simulink model "MagLevNL_wNoise_Lab10_CS"  (Simulink 10.0)
settings: Solver=VariableStepAuto  StartTime=0.0  StopTime=30  MaxStep=1e-4  RelTol=1e-6  AbsTol=1e-6
InitFcn:
  | K_plant = 1.241578125e-3+0.3*(1-2*rand)*1e-3
libraries: cstblocks x1, simulink x1
settings Model: Creator=MENGQI  LastModifiedBy=Santoshi Kulkarni
settings SolverCC: AutoScaleAbsTol=off  InitialStep=1e-7
settings DataIOCC: SaveFormat=Dataset
settings OptimizationCC: LifeSpan=auto
settings DebuggingCC: UnderspecifiedInitializationDetection=Simplified  MergeDetectMultiDrivingBlocksExec=error  SFUnexpectedBacktrackingDiag=error  SFNoUnconditionalDefaultTransitionDiag=error  SFExecutionAtInitializationDiag=warning
settings HardwareCC: ProdBitPerPointer=64  ProdBitPerSizeT=64  ProdBitPerPtrDiffT=64  ProdLargestAtomicFloat=Float  ProdIntDivRoundTo=Zero  ProdEndianess=LittleEndian  ProdWordSize=64  ProdHWDeviceType=Intel->x86-64 (Windows64)
settings ModelReferenceCC: PropagateSignalLabelsOutOfModel=on
settings GRTTargetCC: TargetLangStandard=C99 (ISO)  CombineOutputUpdateFcns=on  GRTInterface=off
settings ConfigComp: CovMetricSettings=dwe  CovHtmlReporting=off  CovSaveCumulativeToWorkspaceVar=off  CovSaveSingleToWorkspaceVar=off

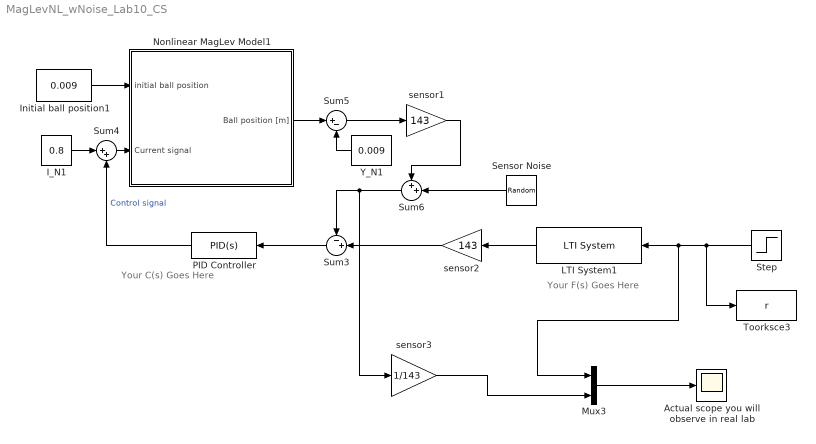
== system MagLevNL_wNoise_Lab10_CS ==
  note: Your F(s) Goes Here
  note: Your C(s) Goes Here
  Actual scope you will observe in real lab : Scope
  I_N1 : Constant  Value=0.8
  Initial ball position1 : Constant  Value=0.009
  LTI System1 : cstblocks/LTI System  sys=tf(5,[1 5])  IC=[]
  Mux3 : Mux  Inputs=2
  Nonlinear MagLev Model1 : Subsystem
  PID Controller : simulink/Continuous/PID Controller  Controller=PID  Form=Parallel  TimeDomain=Continuous-time  SampleTime=-1  IntegratorMethod=Forward Euler  FilterMethod=Forward Euler  ControllerParametersSource=internal  P=-4.45  I=-3.09  D=-0.0532  UseFilter=on  N=1000  TunerSelectOption=Transfer Function Based (PID Tuner App)  InitialConditionSource=internal  InitialConditionForIntegrator=0  InitialConditionForFilter=0  DifferentiatorICPrevScaledInput=0  ExternalReset=none  TrackingMode=off  Kt=1  LimitOutput=off  UpperSaturationLimit=inf  LowerSaturationLimit=-inf  LinearizeAsGain=on  AntiWindupMode=none  Kb=1  POutMin=[]  POutMax=[]  IOutMin=[]  IOutMax=[]  DOutMin=[]  DOutMax=[]  NOutMin=[]  NOutMax=[]  SumOutMin=[]  SumOutMax=[]  SaturationOutMin=[]  SaturationOutMax=[]  PParamMin=[]  PParamMax=[]  IParamMin=[]  IParamMax=[]  DParamMin=[]  DParamMax=[]  NParamMin=[]  NParamMax=[]  KbParamMin=[]  KbParamMax=[]  KtParamMin=[]  KtParamMax=[]  KbOutMin=[]  KbOutMax=[]  KtOutMin=[]  KtOutMax=[]  IntegratorOutMin=[]  IntegratorOutMax=[]  FilterOutMin=[]  FilterOutMax=[]  SumI1OutMin=[]  SumI1OutMax=[]  SumI2OutMin=[]  SumI2OutMax=[]  SumI3OutMin=[]  SumI3OutMax=[]  SumI4OutMin=[]  SumI4OutMax=[]  SumDOutMin=[]  SumDOutMax=[]  DifferentiatorOutMin=[]  DifferentiatorOutMax=[]  FilterDiffOutCoefMin=[]  FilterDiffOutCoefMax=[]  ReciprocalOutMin=[]  ReciprocalOutMax=[]  SumDenOutMin=[]  SumDenOutMax=[]  SumNumOutMin=[]  SumNumOutMax=[]  DivideOutMin=[]  DivideOutMax=[]  IntegratorContinuousStateAttributes=''  IntegratorStateMustResolveToSignalObject=off  IntegratorRTWStateStorageClass=Auto  FilterContinuousStateAttributes=''  FilterStateMustResolveToSignalObject=off  FilterRTWStateStorageClass=Auto  ParallelPVariant=InternalParameters  IdealPVariant=Disabled  IVariant=InternalParameters  DVariant=InternalParameters  IntegratorVariant=Continuous  SatVariant=Disabled  AWVariant=Passthrough  PCopyVariant=Disabled  TRVariant=Disabled  FdbkBlocksVariant=Forward  IdealPFdbkVariant=Disabled  SatFdbkVariant=Disabled  DerivativeFilterVariant=ContFilter  NVariant=InternalParameters  NCopyVariant=Disabled  FilterICVariant=InternalICsFilter  IntegratorICVariant=InternalICs  ExternalResetVariant=Disabled  TRSumVariant=Passthrough  SumFdbkVariant=Disabled  SumVariant=Sum_PID
  Sensor Noise : RandomNumber  Variance=5e-5  SampleTime=0.01
  Step : Step  Time=3  After=0.012  SampleTime=0
  Sum3 : Sum  Inputs=-+|
  Sum4 : Sum  Inputs=|++
  Sum5 : Sum  Inputs=|+-
  Sum6 : Sum  Inputs=++|
  Toorksce3 : ToWorkspace  VariableName=r  SampleTime=0.01
  Y_N1 : Constant  Value=0.009
  sensor1 : Gain  Gain=143
  sensor2 : Gain  Gain=143
  sensor3 : Gain  Gain=1/143
  wires:
  PID Controller/1 -> Sum4/2  "Control signal"
  Step/1 -> LTI System1/1, Mux3/1, Toorksce3/1
  Initial ball position1/1 -> Nonlinear MagLev Model1/1(initial ball position)
  Sum4/1 -> Nonlinear MagLev Model1/2(Current signal)
  I_N1/1 -> Sum4/1
  Nonlinear MagLev Model1/1(Ball position [m]) -> Sum5/1
  Sum5/1 -> sensor1/1
  Y_N1/1 -> Sum5/2
  Sum3/1 -> PID Controller/1
  sensor2/1 -> Sum3/2
  LTI System1/1 -> sensor2/1
  sensor3/1 -> Mux3/2
  sensor1/1 -> Sum6/1
  Sensor Noise/1 -> Sum6/2
  Sum6/1 -> sensor3/1, Sum3/1
  Mux3/1 -> Actual scope you will observe in real lab/1

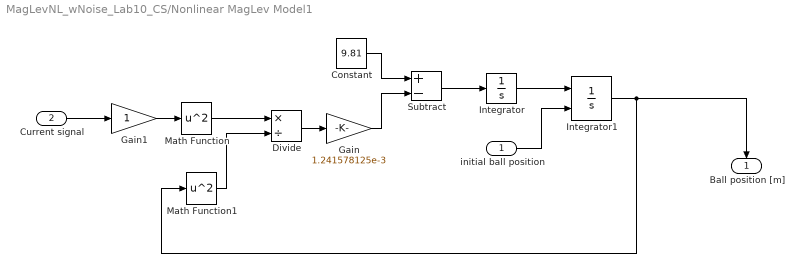
== system MagLevNL_wNoise_Lab10_CS/Nonlinear MagLev Model1 ==
  initial ball position : Inport
  Current signal : Inport  Port=2
  Constant : Constant  Value=9.81
  Divide : Product  Inputs=*/
  Gain : Gain  Gain=1.241578125e-3
  Gain1 : Gain
  Integrator : Integrator
  Integrator1 : Integrator  InitialConditionSource=external
  Math Function : Math  Operator=square  SaturateOnIntegerOverflow=on
  Math Function1 : Math  Operator=square  SaturateOnIntegerOverflow=on
  Subtract : Sum  Inputs=+-
  Ball position [m] : Outport
  wires:
  Gain1/1 -> Math Function/1
  Current signal/1 -> Gain1/1
  initial ball position/1 -> Integrator1/2
  Integrator1/1 -> Math Function1/1, Ball position [m]/1
  Integrator/1 -> Integrator1/1
  Subtract/1 -> Integrator/1
  Gain/1 -> Subtract/2
  Divide/1 -> Gain/1
  Math Function1/1 -> Divide/2
  Math Function/1 -> Divide/1
  Constant/1 -> Subtract/1
